simulink library "sldvdemolib_boundarytest"  (Simulink 7.6)
settings: Solver=ode45  SolverMode=SingleTasking  StartTime=0.0  StopTime=10.0  RelTol=1e-3
libraries: sldvdemolib_boundarytest x1
settings Model: Creator=yito  LastModifiedBy=itoy

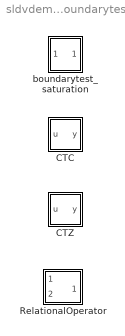
== system sldvdemolib_boundarytest ==
  CTC : Subsystem  mask(Compare To Constant){relop=<=, const=3.0, OutDataTypeStr=uint8, ZeroCross=on}
      mask prompts: relop "Simulink:masks:Operator_MP"; const "Simulink:masks:ConstantValue_MP"; OutDataTypeStr "Simulink:masks:OutputDataType_MP"; ZeroCross "Simulink:masks:EnableZerocrossingDetection_MP"
      mask help: Simulink:masks:CompareToConstant_MD
      mask init:
      | blkName = gcb;
      | 
      | if strcmp(get_param(gcbh,'OutDataTypeStr'),'boolean')
      | 	setValue = 'boolean';
      | else
      | 	setValue = 'fixdt(0, 8)';
      | end
      | 
      | set_param([blkName,'/Compare'],'relop',relop, ...
      | 	'OutDataTypeStr', setValue, 'ZeroCross', ZeroCross);
      | 
      | str = [relop,' C']; %default
      | 
      | const_str = get_param(blkName, 'const');
      | 
      | if isempty(strfind(const_str, ' ')) && isempty(strfind(const_str, ','))
      |     % scalar or single expression
      |     if isempty(str2num(const_str))
      |         %expression
      |         str = [relop, ' ', const_str];
      |     elseif length(const) == 1
      |         str = [relop,' ',num2str(double(const))];
      |     end
      | end
      mask StyleString: popup(==|~=|<|<=|>=|>),edit,popup(uint8|boolean),checkbox
      mask CallbackString: |||sl('zeroCrossEnable', gcbh);
      mask Display: disp(str)
  CTZ : Subsystem  mask(Compare To Zero){relop=<=, OutDataTypeStr=uint8, ZeroCross=on}
      mask prompts: relop "Simulink:masks:Operator_MP"; OutDataTypeStr "Simulink:masks:OutputDataType_MP"; ZeroCross "Simulink:masks:EnableZerocrossingDetection_MP"
      mask help: Simulink:masks:CompareToZero_MD
      mask init:
      | blkName = gcb;
      | 
      | if strcmp(get_param(gcbh,'OutDataTypeStr'),'boolean')
      | 	setValue = 'boolean';
      | else
      |     setValue = 'fixdt(0, 8)';
      | end
      | 
      | set_param([blkName,'/Compare'],'relop',relop, ...
      | 	'OutDataTypeStr', setValue, 'ZeroCross', ZeroCross);
      mask StyleString: popup(==|~=|<|<=|>=|>),popup(uint8|boolean),checkbox
      mask CallbackString: ||sl('zeroCrossEnable', gcbh);
      mask Display: disp([relop,' 0'])
  RelationalOperator : Subsystem  mask{relop=<}
      mask prompts: relop "Relational Operator"
      mask init:
      | set_param([gcb '/relop'],'relop',relop);
      mask Display: disp(relop)
  boundarytest_saturation : Subsystem  mask{UpperLimit=100, LowerLimit=1}
      mask help:
      | Block replacement rule for Saturation block.
      | This block enables you a boundary check.
      mask Display: disp('Saturation\nBoundary Test')

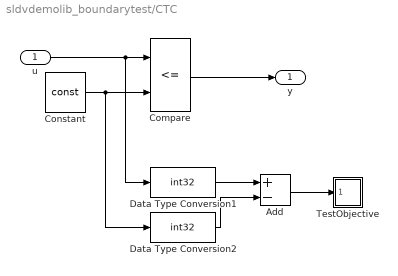
== system sldvdemolib_boundarytest/CTC ==
  u : Inport
  Add : Sum  Inputs=+-  OutDataTypeStr=Inherit: Same as first input
  Compare : RelationalOperator  Operator=<=  OutDataTypeStr=fixdt(0, 8)  InputSameDT=on
  Constant : Constant  DisableCoverage=on  Value=const  OutDataTypeStr=Inherit: Inherit via back propagation
  Data Type Conversion1 : DataTypeConversion  OutDataTypeStr=int32  ConvertRealWorld=Stored Integer (SI)
  Data Type Conversion2 : DataTypeConversion  OutDataTypeStr=int32  ConvertRealWorld=Stored Integer (SI)
  TestObjective : Subsystem  mask(Design Verifier Test Objective){enabled=on, customAVTBlockType=Test Objective, intervals={-1,0,1}, dispValues=on, outEnabled=off}
      mask prompts: enabled "Enable"; customAVTBlockType "Type"; intervals "Values"; dispValues "Display values"; outEnabled "Pass through style (show Outport)"
      mask help:
      | Obtains signal values in Simulink Design Verifier test cases.  The 'Values' parameter specifies the desired input signal values.  Two element vectors specify intervals.  Cell arrays specify lists.  Each list entry might result in a separate test case.
      | Example Values:
      | true
      | {[0 1], 2, [4 5], 6}
      | {Sldv.Interval(-2, -1), Sldv.Point(0), Sldv.Interval(0, 1, '()'), 1}
      mask init:
      | customAVTParams = customAVTBlock(gcb, 'update_from_mask', intervals);
      settings: AttributesFormatString=%<intervals>
      mask Help: helpview(fullfile(docroot,'toolbox','sldv','sldv.map'),'testobjective')
      mask StyleString: checkbox,popup(Test Objective|Proof Objective),edit,checkbox,checkbox
      mask CallbackString: |||customAVTBlock(gcb,'updateDisp');|
      mask Display: image(imread('sldvicon_o_normal.png','BackGroundColor',[1 1 1]),[3 3 19 20]); hide_arrows(true);
  y : Outport
  wires:
  u/1 -> Compare/1, Data Type Conversion1/1
  Constant/1 -> Compare/2, Data Type Conversion2/1
  Compare/1 -> y/1
  Data Type Conversion2/1 -> Add/2
  Data Type Conversion1/1 -> Add/1
  Add/1 -> TestObjective/1(In1)

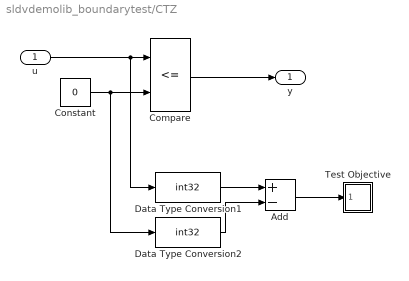
== system sldvdemolib_boundarytest/CTZ ==
  u : Inport
  Add : Sum  Inputs=+-  OutDataTypeStr=Inherit: Same as first input
  Compare : RelationalOperator  Operator=<=  OutDataTypeStr=fixdt(0, 8)  InputSameDT=on
  Constant : Constant  DisableCoverage=on  Value=0  OutDataTypeStr=Inherit: Inherit via back propagation  PreserveConstantTs=on
  Data Type Conversion1 : DataTypeConversion  OutDataTypeStr=int32  ConvertRealWorld=Stored Integer (SI)
  Data Type Conversion2 : DataTypeConversion  OutDataTypeStr=int32  ConvertRealWorld=Stored Integer (SI)
  Test Objective : Subsystem  mask(Design Verifier Test Objective){enabled=on, customAVTBlockType=Test Objective, intervals={-1,0,1}, dispValues=on, outEnabled=off}
      mask prompts: enabled "Enable"; customAVTBlockType "Type"; intervals "Values"; dispValues "Display values"; outEnabled "Pass through style (show Outport)"
      mask help:
      | Obtains signal values in Simulink Design Verifier test cases.  The 'Values' parameter specifies the desired input signal values.  Two element vectors specify intervals.  Cell arrays specify lists.  Each list entry might result in a separate test case.
      | Example Values:
      | true
      | {[0 1], 2, [4 5], 6}
      | {Sldv.Interval(-2, -1), Sldv.Point(0), Sldv.Interval(0, 1, '()'), 1}
      mask init:
      | customAVTParams = customAVTBlock(gcb, 'update_from_mask', intervals);
      settings: AttributesFormatString=%<intervals>
      mask Help: helpview(fullfile(docroot,'toolbox','sldv','sldv.map'),'testobjective')
      mask StyleString: checkbox,popup(Test Objective|Proof Objective),edit,checkbox,checkbox
      mask CallbackString: |||customAVTBlock(gcb,'updateDisp');|
      mask Display: image(imread('sldvicon_o_normal.png','BackGroundColor',[1 1 1]),[3 3 19 20]); hide_arrows(true);
  y : Outport
  wires:
  Constant/1 -> Compare/2, Data Type Conversion2/1
  u/1 -> Compare/1, Data Type Conversion1/1
  Compare/1 -> y/1
  Data Type Conversion2/1 -> Add/2
  Data Type Conversion1/1 -> Add/1
  Add/1 -> Test Objective/1(In1)

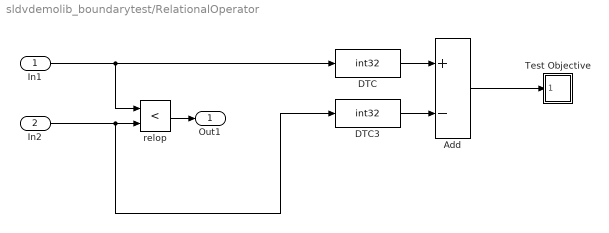
== system sldvdemolib_boundarytest/RelationalOperator ==
  In1 : Inport
  In2 : Inport  Port=2
  Add : Sum  Inputs=+-  OutDataTypeStr=int32
  DTC : DataTypeConversion  OutDataTypeStr=int32  ConvertRealWorld=Stored Integer (SI)
  DTC3 : DataTypeConversion  OutDataTypeStr=int32  ConvertRealWorld=Stored Integer (SI)
  Test Objective : Subsystem  mask(Design Verifier Test Objective){enabled=on, customAVTBlockType=Test Objective, intervals={-1,0,1}, dispValues=on, outEnabled=off}
      mask prompts: enabled "Enable"; customAVTBlockType "Type"; intervals "Values"; dispValues "Display values"; outEnabled "Pass through style (show Outport)"
      mask help:
      | Obtains signal values in Simulink Design Verifier test cases.  The 'Values' parameter specifies the desired input signal values.  Two element vectors specify intervals.  Cell arrays specify lists.  Each list entry might result in a separate test case.
      | Example Values:
      | true
      | {[0 1], 2, [4 5], 6}
      | {Sldv.Interval(-2, -1), Sldv.Point(0), Sldv.Interval(0, 1, '()'), 1}
      mask init:
      | customAVTParams = customAVTBlock(gcb, 'update_from_mask', intervals);
      settings: AttributesFormatString=%<intervals>
      mask Help: helpview(fullfile(docroot,'toolbox','sldv','sldv.map'),'testobjective')
      mask StyleString: checkbox,popup(Test Objective|Proof Objective),edit,checkbox,checkbox
      mask CallbackString: |||customAVTBlock(gcb,'updateDisp');|
      mask Display: image(imread('sldvicon_o_normal.png','BackGroundColor',[1 1 1]),[3 3 19 20]); hide_arrows(true);
  relop : RelationalOperator  Operator=<  OutDataTypeStr=boolean
  Out1 : Outport
  wires:
  In1/1 -> relop/1, DTC/1
  relop/1 -> Out1/1
  In2/1 -> relop/2, DTC3/1
  DTC/1 -> Add/1
  DTC3/1 -> Add/2
  Add/1 -> Test Objective/1(In1)

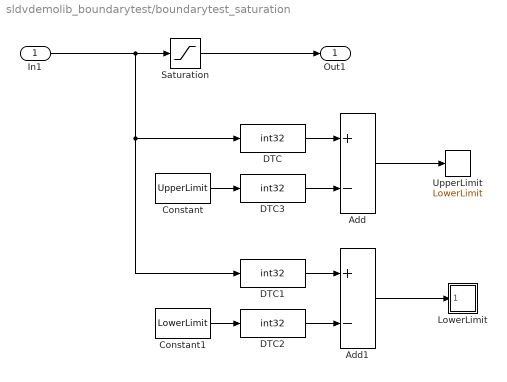
== system sldvdemolib_boundarytest/boundarytest_saturation ==
  In1 : Inport
  Add : Sum  Inputs=+-  OutDataTypeStr=int32
  Add1 : Sum  Inputs=+-  OutDataTypeStr=int32
  Constant : Constant  Value=UpperLimit
  Constant1 : Constant  Value=LowerLimit
  DTC{,1..3} (4 alike) : DataTypeConversion  OutDataTypeStr=int32  ConvertRealWorld=Stored Integer (SI)
  LowerLimit : Subsystem  mask(Design Verifier Test Objective){enabled=on, customAVTBlockType=Test Objective, intervals={-1,0,1}, dispValues=on, outEnabled=off}
      mask prompts: enabled "Enable"; customAVTBlockType "Type"; intervals "Values"; dispValues "Display values"; outEnabled "Pass through style (show Outport)"
      mask help:
      | Obtains signal values in Simulink Design Verifier test cases.  The 'Values' parameter specifies the desired input signal values.  Two element vectors specify intervals.  Cell arrays specify lists.  Each list entry might result in a separate test case.
      | Example Values:
      | true
      | {[0 1], 2, [4 5], 6}
      | {Sldv.Interval(-2, -1), Sldv.Point(0), Sldv.Interval(0, 1, '()'), 1}
      mask init:
      | customAVTParams = customAVTBlock(gcb, 'update_from_mask', intervals);
      settings: AttributesFormatString=%<intervals>
      mask Help: helpview(fullfile(docroot,'toolbox','sldv','sldv.map'),'testobjective')
      mask StyleString: checkbox,popup(Test Objective|Proof Objective),edit,checkbox,checkbox
      mask CallbackString: |||customAVTBlock(gcb,'updateDisp');|
      mask Display: image(imread('sldvicon_o_normal.png','BackGroundColor',[1 1 1]),[3 3 19 20]); hide_arrows(true);
  Saturation : Saturate  UpperLimit=UpperLimit  LowerLimit=LowerLimit
  UpperLimit : sldvdemolib_boundarytest/boundarytest_saturation/LowerLimit  SystemSampleTime=-1  enabled=on  customAVTBlockType=Test Objective  intervals={-1,0,1}  dispValues=on  outEnabled=off
      settings: AttributesFormatString=%<intervals>
  Out1 : Outport
  wires:
  In1/1 -> Saturation/1, DTC/1, DTC1/1
  Saturation/1 -> Out1/1
  Add/1 -> UpperLimit/1
  Constant/1 -> DTC3/1
  DTC/1 -> Add/1
  Add1/1 -> LowerLimit/1(In1)
  Constant1/1 -> DTC2/1
  DTC1/1 -> Add1/1
  DTC2/1 -> Add1/2
  DTC3/1 -> Add/2

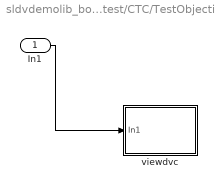
== system sldvdemolib_boundarytest/CTC/TestObjective ==
  In1 : Inport
  viewdvc : Subsystem  TreatAsAtomicUnit=on  SimViewingDevice=on  mask(VerificationSubsystem){}
      mask init:
      | sldvsubsys('maskInit');
  wires:
  In1/1 -> viewdvc/1(In1)

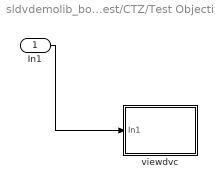
== system sldvdemolib_boundarytest/CTZ/Test Objective ==
  In1 : Inport
  viewdvc : Subsystem  TreatAsAtomicUnit=on  SimViewingDevice=on  mask(VerificationSubsystem){}
      mask init:
      | sldvsubsys('maskInit');
  wires:
  In1/1 -> viewdvc/1(In1)

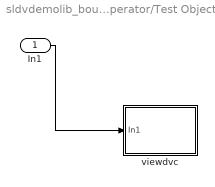
== system sldvdemolib_boundarytest/RelationalOperator/Test Objective ==
  In1 : Inport
  viewdvc : Subsystem  TreatAsAtomicUnit=on  SimViewingDevice=on  mask(VerificationSubsystem){}
      mask init:
      | sldvsubsys('maskInit');
  wires:
  In1/1 -> viewdvc/1(In1)

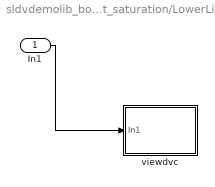
== system sldvdemolib_boundarytest/boundarytest_saturation/LowerLimit ==
  In1 : Inport
  viewdvc : Subsystem  TreatAsAtomicUnit=on  SimViewingDevice=on  mask(VerificationSubsystem){}
      mask init:
      | sldvsubsys('maskInit');
  wires:
  In1/1 -> viewdvc/1(In1)

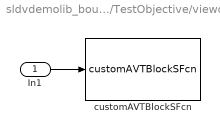
== system sldvdemolib_boundarytest/CTC/TestObjective/viewdvc ==
  In1 : Inport
  customAVTBlockSFcn : S-Function  FunctionName=customAVTBlockSFcn  EnableBusSupport=off
  wires:
  In1/1 -> customAVTBlockSFcn/1

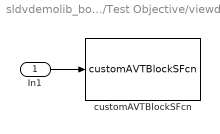
== system sldvdemolib_boundarytest/CTZ/Test Objective/viewdvc ==
  In1 : Inport
  customAVTBlockSFcn : S-Function  FunctionName=customAVTBlockSFcn  EnableBusSupport=off
  wires:
  In1/1 -> customAVTBlockSFcn/1

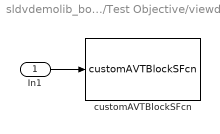
== system sldvdemolib_boundarytest/RelationalOperator/Test Objective/viewdvc ==
  In1 : Inport
  customAVTBlockSFcn : S-Function  FunctionName=customAVTBlockSFcn  EnableBusSupport=off
  wires:
  In1/1 -> customAVTBlockSFcn/1

== system sldvdemolib_boundarytest/boundarytest_saturation/LowerLimit/viewdvc ==
  In1 : Inport
  customAVTBlockSFcn : S-Function  FunctionName=customAVTBlockSFcn  EnableBusSupport=off
  wires:
  In1/1 -> customAVTBlockSFcn/1
